simulink model "First_Order_system"  (R2014a)
settings: Solver=ode45  StartTime=0.0  StopTime=120  RelTol=1e-3
model workspace: external: MATLAB File D:\Working\Modern Control Engineering\Study\Adaptive Control\Adaptive Controllers\Model Reference Adatptive Controller MRAC\First Order system\source.m (data not in the file)
values from neighbouring files (symbols this model uses):
  a = 2.0636    [source.m]
  am = 0.6159    [MITrule.m]    (also in mit.m = 0.8282; mitrule2.m = 0.6065; mr2.m; source.m = 4.1271)
  b = 5.7072    [source.m]
  bm = 2.193    [MITrule.m]    (also in mit.m = 0.1718; mitrule2.m = 0.3935; mr2.m; source.m = 11.4144)
  gamma = 60    [source.m]
settings Model: Creator=Ahmed ElTahan  LastModifiedBy=Ahmed ElTahan

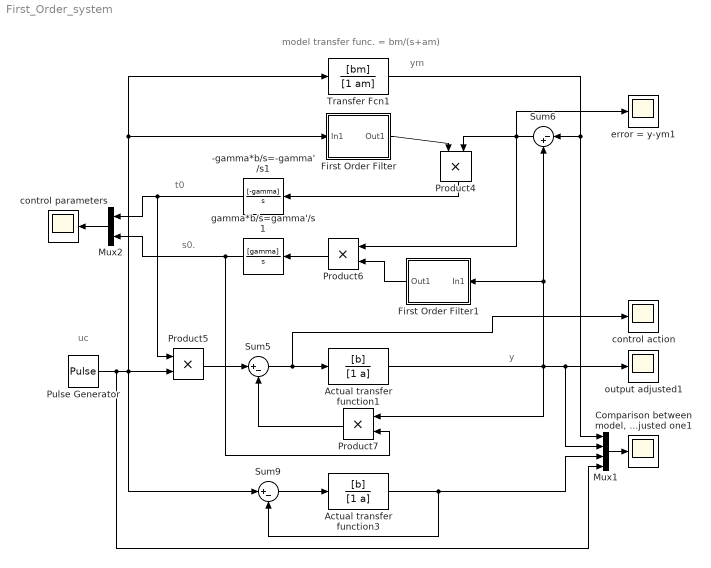
== system First_Order_system ==
  note: s0.
  note: t0
  note: uc
  note: y
  note: ym
  note: model transfer func. = bm/(s+am)
  -gamma*b/s=-gamma'/s1 : TransferFcn  Numerator=[-gamma]  Denominator=[1 0]
  Actual transfer function1 : TransferFcn  Numerator=[b]  Denominator=[1 a]
  Actual transfer function3 : TransferFcn  Numerator=[b]  Denominator=[1 a]
  "Comparison between model, adjusted and not ajusted one1" : Scope
      settings: SaveName=output
  "First Order Filter " : Subsystem
  First Order Filter1 : Subsystem
  Mux1 : Mux
  Mux2 : Mux  Inputs=2
  Product{4..7} (4 alike) : Product
  Pulse Generator : DiscretePulseGenerator  PulseType=Time based  Period=20  PulseWidth=50
  Sum5 : Sum  Inputs=|+-
  Sum6 : Sum  Inputs=|-+
  Sum9 : Sum  Inputs=|+-
  Transfer Fcn1 : TransferFcn  Numerator=[bm]  Denominator=[1 am]
  control parameters : Scope
      settings: SaveName=ContParam
  control action : Scope
      settings: SaveName=u
  error = y-ym1 : Scope
      settings: SaveName=err
  gamma*b/s=gamma'/s1 : TransferFcn  Numerator=[gamma]  Denominator=[1 0]
  output adjusted1 : Scope
      settings: SaveName=ScopeData7
  wires:
  Product5/1 -> Sum5/1
  Product7/1 -> Sum5/2
  Sum5/1 -> control action/1, Actual transfer function1/1
  Actual transfer function1/1 -> Product7/1, Mux1/2, output adjusted1/1, First Order Filter1/1(In1), Sum6/2
  Transfer Fcn1/1 -> Sum6/1, Mux1/1
  Product4/1 -> -gamma*b/s=-gamma'/s1/1
  -gamma*b/s=-gamma'/s1/1 -> Mux2/1, Product5/1
  Sum6/1 -> error = y-ym1/1, Product6/1, Product4/2
  Product6/1 -> gamma*b/s=gamma'/s1/1
  gamma*b/s=gamma'/s1/1 -> Mux2/2, Product7/2
  Sum9/1 -> Actual transfer function3/1
  Actual transfer function3/1 -> Sum9/2, Mux1/3
  Pulse Generator/1 -> Mux1/4, Sum9/1, Product5/2, "First Order Filter "/1(In1), Transfer Fcn1/1
  "First Order Filter "/1(Out1) -> Product4/1
  First Order Filter1/1(Out1) -> Product6/2
  Mux1/1 -> "Comparison between model, adjusted and not ajusted one1"/1
  Mux2/1 -> control parameters/1

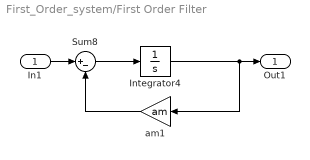
== system First_Order_system/First Order Filter  ==
  In1 : Inport
  Integrator4 : Integrator
  Sum8 : Sum  Inputs=|+-
  am1 : Gain  Gain=am
  Out1 : Outport
  wires:
  Sum8/1 -> Integrator4/1
  am1/1 -> Sum8/2
  Integrator4/1 -> Out1/1, am1/1
  In1/1 -> Sum8/1

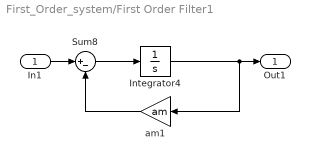
== system First_Order_system/First Order Filter1 ==
  In1 : Inport
  Integrator4 : Integrator
  Sum8 : Sum  Inputs=|+-
  am1 : Gain  Gain=am
  Out1 : Outport
  wires:
  Sum8/1 -> Integrator4/1
  am1/1 -> Sum8/2
  Integrator4/1 -> Out1/1, am1/1
  In1/1 -> Sum8/1
